simulink model "final"  (R2014a)
settings: Solver=ode45  StartTime=0.0  StopTime=0.01  RelTol=1e-3
libraries: powerlib x52
settings Model: Creator=ANSI  LastModifiedBy=SAIKUMAR
settings OptimizationCC: ExpressionDepthLimit=2147483647
settings DebuggingCC: UnderspecifiedInitializationDetection=Classic  StateNameClashWarn=warning
settings GRTTargetCC: CombineOutputUpdateFcns=off  GRTInterface=on

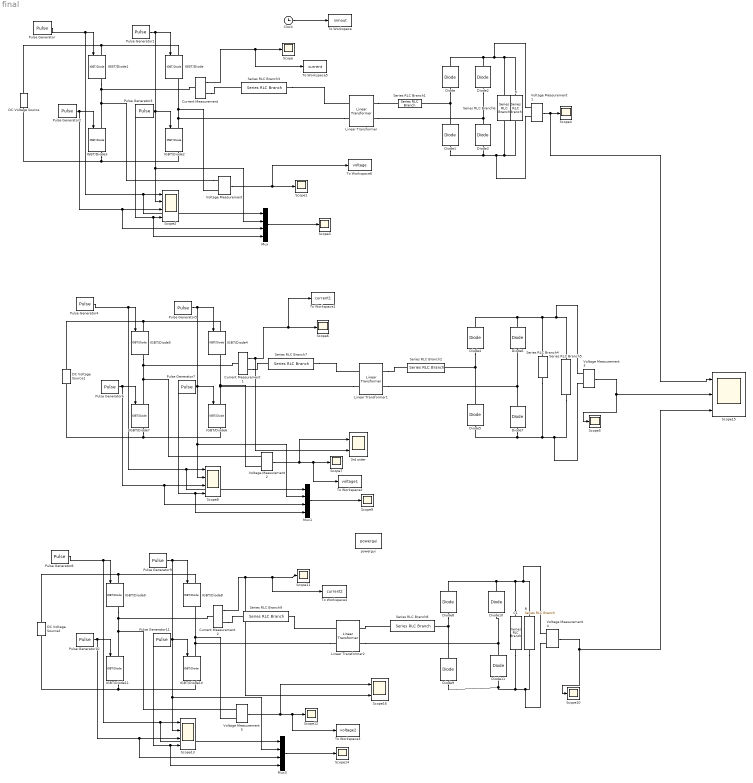
== system final ==
  " R" : powerlib/Elements/Series RLC Branch  LConnTagsString=__new0  RConnTagsString=__new0  BranchType=R  Resistance=20  Inductance=39e-6  SetiL0=off  InitialCurrent=0  Capacitance=1e-6  Setx0=off  InitialVoltage=0  Measurements=None
  3rd order : Scope  NumInputPorts=2
      settings: TickLabels=on  TimeRange=0.01  YMin=-500~-5  YMax=500~5  SaveName=ScopeData6  SampleInput=on
  C1 : powerlib/Elements/Series RLC Branch  LConnTagsString=__new0  RConnTagsString=__new0  BranchType=C  Resistance=0.1  Inductance=1e-3  SetiL0=off  InitialCurrent=0  Capacitance=27e-6  Setx0=off  InitialVoltage=0  Measurements=None
  Clock : Clock
  Current Measurement : powerlib/Measurements/Current Measurement  PhasorSimulation=off  OutputType=Complex  PSBequivalent=0
  Current Measurement1 : powerlib/Measurements/Current Measurement  PhasorSimulation=off  OutputType=Complex  PSBequivalent=0
  Current Measurement2 : powerlib/Measurements/Current Measurement  PhasorSimulation=off  OutputType=Complex  PSBequivalent=0
  DC Voltage Source : powerlib/Electrical Sources/DC Voltage Source  Amplitude=90  Measurements=None
  DC Voltage Source1 : powerlib/Electrical Sources/DC Voltage Source  Amplitude=90  Measurements=None
  DC Voltage Source2 : powerlib/Electrical Sources/DC Voltage Source  Amplitude=90  Measurements=None
  Diode{,1..11} (12 alike) : powerlib/Power Electronics/Diode  Ron=0.001  Lon=0  Vf=0.8  IC=0  UseSnubber=off  Rs=500  Cs=250e-9  Measurements=off
  IGBT/Diode{,1..11} (12 alike) : powerlib/Power Electronics/IGBT//Diode  Ron=1e-3  Rs=1e5  Cs=inf  Measurements=on
  Linear Transformer : powerlib/Elements/Linear Transformer  UNITS=SI  NominalPower=[ 2.5e3 60 ]  winding1=[100 0.1 39e-6]  winding2=[180 0.2 149e-6]  ThreeWindings=off  winding3=[3.15e+005 0.7938 0.00012032]  RmLm=[1 16e-6]  Measurements=None  DataType=on
  Linear Transformer1 : powerlib/Elements/Linear Transformer  UNITS=SI  NominalPower=[ 2.5e3 60 ]  winding1=[90 0.1 39e-6]  winding2=[350 0.2 149e-6]  ThreeWindings=off  winding3=[3.15e+005 79380 8422.5]  RmLm=[1 16e-6]  Measurements=None  DataType=on
  Linear Transformer2 : powerlib/Elements/Linear Transformer  UNITS=SI  NominalPower=[ 2.5e3 60 ]  winding1=[90 0.1 39e-6]  winding2=[250 0.2 149e-6]  ThreeWindings=off  winding3=[3.15e+005 0.7938 0.084225]  RmLm=[1 16e-6]  Measurements=None  DataType=on
  Mux : Mux
  Mux1 : Mux
  Mux3 : Mux
  Pulse Generator : DiscretePulseGenerator  PulseType=Time based  Amplitude=10  Period=23.8e-6  PulseWidth=45.79
  Pulse Generator1 : DiscretePulseGenerator  PulseType=Time based  Amplitude=10  Period=23.8e-6  PulseWidth=45.79  PhaseDelay=21.486e-6
  Pulse Generator10 : DiscretePulseGenerator  PulseType=Time based  Amplitude=10  Period=119.04e-6  PulseWidth=49.16  PhaseDelay=60.52e-6
  Pulse Generator11 : DiscretePulseGenerator  PulseType=Time based  Amplitude=10  Period=119.04e-6  PulseWidth=49.16
  Pulse Generator2 : DiscretePulseGenerator  PulseType=Time based  Amplitude=10  Period=23.8e-6  PulseWidth=45.79  PhaseDelay=13.22e-6
  Pulse Generator3 : DiscretePulseGenerator  PulseType=Time based  Amplitude=10  Period=23.8e-6  PulseWidth=45.79  PhaseDelay=8.26e-6
  Pulse Generator4 : DiscretePulseGenerator  PulseType=Time based  Amplitude=10  Period=71.42e-6  PulseWidth=48.599
  Pulse Generator5 : DiscretePulseGenerator  PulseType=Time based  Amplitude=10  Period=71.42e-6  PulseWidth=48.599  PhaseDelay=44.64e-6
  Pulse Generator6 : DiscretePulseGenerator  PulseType=Time based  Amplitude=10  Period=71.42e-6  PulseWidth=48.599  PhaseDelay=39.68e-6
  Pulse Generator7 : DiscretePulseGenerator  PulseType=Time based  Amplitude=10  Period=71.42e-6  PulseWidth=48.599  PhaseDelay=4.96e-6
  Pulse Generator8 : DiscretePulseGenerator  PulseType=Time based  Amplitude=10  Period=119.04e-6  PulseWidth=49.16
  Pulse Generator9 : DiscretePulseGenerator  PulseType=Time based  Amplitude=10  Period=119.04e-6  PulseWidth=49.16  PhaseDelay=60.52e-6
  R : powerlib/Elements/Series RLC Branch  LConnTagsString=__new0  RConnTagsString=__new0  BranchType=R  Resistance=25  Inductance=10e-  SetiL0=off  InitialCurrent=0  Capacitance=10e-6  Setx0=off  InitialVoltage=0  Measurements=None
  Scope{,1,3..7,9..12,14} (12 alike) : Scope
      Scope settings: YMin=-200  YMax=200
      Scope1 settings: TickLabels=on  TimeRange=0.01  YMin=-500  YMax=500  SampleInput=on
      Scope10 settings: TickLabels=on  TimeRange=0.001  YMin=0  YMax=50  SaveName=ScopeData11  SampleInput=on
      Scope11 settings: YMin=-1  YMax=2  SaveName=ScopeData12
      Scope12 settings: TickLabels=on  TimeRange=0.001  YMin=-500  YMax=500  SaveName=ScopeData13  SampleInput=on
      Scope14 settings: TickLabels=on  TimeRange=0.01  YMin=-50  YMax=50  SaveName=ScopeData15  SampleInput=on
      Scope3 settings: TickLabels=on  TimeRange=0.01  YMin=-50  YMax=50  SaveName=ScopeData3  SampleInput=on
      Scope4 settings: TickLabels=on  TimeRange=0.001  YMin=0  YMax=50  SaveName=ScopeData4  SampleInput=on
      Scope5 settings: TickLabels=on  TimeRange=0.01  YMin=0  YMax=50  SaveName=ScopeData5  SampleInput=on
      Scope6 settings: YMin=-20  YMax=20  SaveName=ScopeData7
      Scope7 settings: TickLabels=on  TimeRange=0.01  YMin=-1000  YMax=1000  SaveName=ScopeData8  SampleInput=on
      Scope9 settings: TickLabels=on  TimeRange=0.01  YMin=-50  YMax=50  SaveName=ScopeData10  SampleInput=on
  Scope13 : Scope  NumInputPorts=4
      settings: YMin=-20~-20~-20~-20  YMax=20~20~20~20  SaveName=ScopeData14
  Scope15 : Scope  NumInputPorts=3
      settings: TickLabels=on  TimeRange=0.001  YMin=0~-5~-5  YMax=50~5~5  SaveName=ScopeData17  SampleInput=on
  Scope16 : Scope  NumInputPorts=2
      settings: TickLabels=on  TimeRange=0.001  YMin=-500~-5  YMax=500~5  SaveName=ScopeData16  SampleInput=on
  Scope2 : Scope  NumInputPorts=4
      settings: YMin=-20~-20~-20~-20  YMax=20~20~20~20  SaveName=ScopeData2
  Scope8 : Scope  NumInputPorts=4
      settings: YMin=-20~-20~-20~-20  YMax=20~20~20~20  SaveName=ScopeData9
  Series RLC Branch1 : powerlib/Elements/Series RLC Branch  LConnTagsString=__new0  RConnTagsString=__new0  BranchType=C  Resistance=0.1  Inductance=1e-3  SetiL0=off  InitialCurrent=0  Capacitance=0.09e-6  Setx0=off  InitialVoltage=0  Measurements=None
  Series RLC Branch2 : powerlib/Elements/Series RLC Branch  LConnTagsString=__new0  RConnTagsString=__new0  BranchType=C  Resistance=0.1  Inductance=1e-3  SetiL0=off  InitialCurrent=0  Capacitance=0.09e-6  Setx0=off  InitialVoltage=0  Measurements=None
  Series RLC Branch3 : powerlib/Elements/Series RLC Branch  LConnTagsString=__new0  RConnTagsString=__new0  BranchType=C  Resistance=0.1  Inductance=1e-3  SetiL0=off  InitialCurrent=0  Capacitance=0.36e-6  Setx0=off  InitialVoltage=0  Measurements=None
  Series RLC Branch4 : powerlib/Elements/Series RLC Branch  LConnTagsString=__new0  RConnTagsString=__new0  BranchType=C  Resistance=0.1  Inductance=1e-3  SetiL0=off  InitialCurrent=0  Capacitance=25e-6  Setx0=off  InitialVoltage=0  Measurements=None
  Series RLC Branch5 : powerlib/Elements/Series RLC Branch  LConnTagsString=__new0  RConnTagsString=__new0  BranchType=R  Resistance=20  Inductance=39e-6  SetiL0=off  InitialCurrent=0  Capacitance=1e-6  Setx0=off  InitialVoltage=0  Measurements=None
  Series RLC Branch6 : powerlib/Elements/Series RLC Branch  LConnTagsString=__new0  RConnTagsString=__new0  BranchType=C  Resistance=20  Inductance=10e-  SetiL0=off  InitialCurrent=0  Capacitance=30e-6  Setx0=off  InitialVoltage=0  Measurements=None
  Series RLC Branch7 : powerlib/Elements/Series RLC Branch  LConnTagsString=__new0  RConnTagsString=__new0  BranchType=C  Resistance=0.1  Inductance=1e-3  SetiL0=off  InitialCurrent=0  Capacitance=0.36e-6  Setx0=off  InitialVoltage=0  Measurements=None
  Series RLC Branch8 : powerlib/Elements/Series RLC Branch  LConnTagsString=__new0  RConnTagsString=__new0  BranchType=C  Resistance=0.1  Inductance=1e-3  SetiL0=off  InitialCurrent=0  Capacitance=0.09e-6  Setx0=off  InitialVoltage=0  Measurements=None
  Series RLC Branch9 : powerlib/Elements/Series RLC Branch  LConnTagsString=__new0  RConnTagsString=__new0  BranchType=C  Resistance=0.1  Inductance=1e-3  SetiL0=off  InitialCurrent=0  Capacitance=0.36e-6  Setx0=off  InitialVoltage=0  Measurements=None
  To Workspace : ToWorkspace  VariableName=simout  SampleTime=-1
  To Workspace1 : ToWorkspace  VariableName=current1  SampleTime=-1
  To Workspace2 : ToWorkspace  VariableName=voltage1  SampleTime=-1
  To Workspace3 : ToWorkspace  VariableName=voltage2  SampleTime=-1
  To Workspace4 : ToWorkspace  VariableName=current2  SampleTime=-1
  To Workspace5 : ToWorkspace  VariableName=current  SampleTime=-1
  To Workspace6 : ToWorkspace  VariableName=voltage  SampleTime=-1
  Voltage Measurement{,1..5} (6 alike) : powerlib/Measurements/Voltage Measurement  PhasorSimulation=off  OutputType=Complex  PSBequivalent=0
  powergui : powerlib/powergui  Priority=1  SimulationMode=Continuous  SolverType=Tustin  SampleTime=50e-6  frequency=60  SPID=off  DisableSnubberDevices=off  DisableRonSwitches=off  DisableVfSwitches=off  SwTol=0  Interpol=off  DisplayEquations=off  Ts=0  methode=off  frequencyindice=0  Pbase=100e6  ErrMax=1e-4  Iterations=50  UnitsV=kV  UnitsW=MW  FunctionMessages=off  echomessages=off  HookPort=off  EnableUseOfTLC=off  x0status=blocks  RestoreLinks=warning  ResistiveCurrentMeasurement=off  Frange=[0:2:500]  Ylog=off  Xlog=on  ShowGrid=off  save=off  variable=ZData  structure=0  ZoomFFT=on  StartTime=0.0  cycles=1  DisplayStyle=1  fundamental=60  FreqAxis=off  MaxFrequency=1000  frequencyindicesteady=1  RmsSteady=1  display=off
  wires:
  Pulse Generator/1 -> IGBT/Diode1/1, Scope2/1, Mux/1
  Pulse Generator1/1 -> IGBT/Diode/1, Scope2/2, Mux/2
  Pulse Generator2/1 -> IGBT/Diode3/1, Scope2/3, Mux/3
  Pulse Generator3/1 -> IGBT/Diode2/1, Scope2/4, Mux/4
  Current Measurement/1 -> Scope/1, To Workspace5/1
  Voltage Measurement/1 -> To Workspace6/1, Scope1/1
  Mux/1 -> Scope3/1
  Clock/1 -> To Workspace/1
  Voltage Measurement1/1 -> Scope4/1, Scope15/1
  Pulse Generator4/1 -> IGBT/Diode5/1, Scope8/1, Mux1/1
  Pulse Generator5/1 -> IGBT/Diode4/1, Scope8/2, Mux1/2
  Pulse Generator6/1 -> IGBT/Diode7/1, Scope8/3, Mux1/3
  Pulse Generator7/1 -> IGBT/Diode6/1, Scope8/4, Mux1/4
  Current Measurement1/1 -> 3rd order/2, Scope6/1, To Workspace1/1
  Voltage Measurement2/1 -> 3rd order/1, Scope7/1, To Workspace2/1
  Mux1/1 -> Scope9/1
  Voltage Measurement3/1 -> Scope5/1, Scope15/2
  Pulse Generator8/1 -> IGBT/Diode9/1, Scope13/1, Mux3/1
  Pulse Generator9/1 -> IGBT/Diode8/1, Scope13/2, Mux3/2
  Pulse Generator10/1 -> IGBT/Diode11/1, Scope13/3, Mux3/3
  Pulse Generator11/1 -> IGBT/Diode10/1, Scope13/4, Mux3/4
  Current Measurement2/1 -> Scope16/2, Scope11/1, To Workspace4/1
  Voltage Measurement5/1 -> Scope16/1, Scope12/1, To Workspace3/1
  Mux3/1 -> Scope14/1
  Voltage Measurement4/1 -> Scope10/1, Scope15/3
  connections:
  Voltage Measurement/LConn1 -- IGBT/Diode3/LConn1 -- IGBT/Diode1/RConn1 -- Current Measurement/LConn1
  Linear Transformer/LConn2 -- IGBT/Diode/RConn1 -- Voltage Measurement/LConn2 -- IGBT/Diode2/LConn1
  IGBT/Diode1/LConn1 -- IGBT/Diode/LConn1 -- DC Voltage Source/RConn1
  IGBT/Diode3/RConn1 -- IGBT/Diode2/RConn1 -- DC Voltage Source/LConn1
  Series RLC Branch1/LConn1 -- Diode/LConn1 -- Diode1/RConn1
  Linear Transformer/RConn2 -- Diode2/LConn1 -- Diode3/RConn1
  Series RLC Branch6/RConn1 -- R/RConn1 -- Diode2/RConn1 -- Diode/RConn1 -- Voltage Measurement1/LConn1
  Voltage Measurement1/LConn2 -- R/LConn1 -- Series RLC Branch6/LConn1 -- Diode1/LConn1 -- Diode3/LConn1
  Series RLC Branch3/LConn1 -- Linear Transformer/LConn1
  Current Measurement/RConn1 -- Series RLC Branch3/RConn1
  Linear Transformer/RConn1 -- Series RLC Branch1/RConn1
  IGBT/Diode5/RConn1 -- Current Measurement1/LConn1 -- Voltage Measurement2/LConn1 -- IGBT/Diode7/LConn1
  Linear Transformer1/LConn2 -- IGBT/Diode6/LConn1 -- Voltage Measurement2/LConn2 -- IGBT/Diode4/RConn1
  IGBT/Diode5/LConn1 -- IGBT/Diode4/LConn1 -- DC Voltage Source1/RConn1
  IGBT/Diode7/RConn1 -- IGBT/Diode6/RConn1 -- DC Voltage Source1/LConn1
  Series RLC Branch2/LConn1 -- Diode4/LConn1 -- Diode5/RConn1
  Linear Transformer1/RConn2 -- Diode6/LConn1 -- Diode7/RConn1
  Voltage Measurement3/LConn2 -- Series RLC Branch5/RConn1 -- Series RLC Branch4/RConn1 -- Diode5/LConn1 -- Diode7/LConn1
  Series RLC Branch4/LConn1 -- Series RLC Branch5/LConn1 -- Voltage Measurement3/LConn1 -- Diode4/RConn1 -- Diode6/RConn1
  Current Measurement1/RConn1 -- Series RLC Branch7/RConn1
  Series RLC Branch7/LConn1 -- Linear Transformer1/LConn1
  Linear Transformer1/RConn1 -- Series RLC Branch2/RConn1
  Current Measurement2/LConn1 -- IGBT/Diode9/RConn1 -- Voltage Measurement5/LConn1 -- IGBT/Diode11/LConn1
  Linear Transformer2/LConn2 -- IGBT/Diode10/LConn1 -- Voltage Measurement5/LConn2 -- IGBT/Diode8/RConn1
  DC Voltage Source2/RConn1 -- IGBT/Diode9/LConn1 -- IGBT/Diode8/LConn1
  DC Voltage Source2/LConn1 -- IGBT/Diode11/RConn1 -- IGBT/Diode10/RConn1
  Series RLC Branch8/LConn1 -- Diode8/LConn1 -- Diode9/RConn1
  Linear Transformer2/RConn2 -- Diode10/LConn1 -- Diode11/RConn1
  C1/LConn1 -- " R"/LConn1 -- Voltage Measurement4/LConn1 -- Diode8/RConn1 -- Diode10/RConn1
  Voltage Measurement4/LConn2 -- " R"/RConn1 -- C1/RConn1 -- Diode9/LConn1 -- Diode11/LConn1
  Linear Transformer2/RConn1 -- Series RLC Branch8/RConn1
  Series RLC Branch9/LConn1 -- Linear Transformer2/LConn1
  Current Measurement2/RConn1 -- Series RLC Branch9/RConn1
